simulink model "ResponseOfOpenLoopSecondOrderSystemForVariousGain"  (R2021a)
settings: Solver=VariableStepAuto  StartTime=0.0  StopTime=10.0  RelTol=1e-3
settings Model: Creator=soumy  LastModifiedBy=soumy

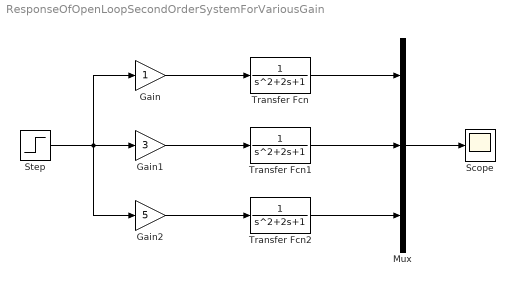
== system ResponseOfOpenLoopSecondOrderSystemForVariousGain ==
  Gain : Gain
  Gain1 : Gain  Gain=3
  Gain2 : Gain  Gain=5
  Mux : Mux  Inputs=3
  Scope : Scope
  Step : Step  SampleTime=0
  Transfer Fcn : TransferFcn
  Transfer Fcn1 : TransferFcn
  Transfer Fcn2 : TransferFcn
  wires:
  Transfer Fcn1/1 -> Mux/2
  Transfer Fcn/1 -> Mux/1
  Transfer Fcn2/1 -> Mux/3
  Gain2/1 -> Transfer Fcn2/1
  Gain1/1 -> Transfer Fcn1/1
  Gain/1 -> Transfer Fcn/1
  Step/1 -> Gain/1, Gain1/1, Gain2/1
  Mux/1 -> Scope/1
